simulink model "suspmod"  (Simulink 8.9)
settings: Solver=FixedStepAuto  StartTime=0.0  StopTime=50  FixedStep=0.01  RelTol=1e-3  AbsTol=1e-6
values from neighbouring files (symbols this model uses):
  m1 = 1    [fcn1.m]
  m2 = 1    [fcn1.m]
undefined symbols (not defined in the file or in its folder): b1, b2, k1, k2
settings Model: SuppressorTable=22 serialization::archive 11 0 6 0 0 0 11 0  Creator=Rick  LastModifiedBy=nikhil
settings DataIOCC: LimitDataPoints=off  SignalLoggingSaveFormat=Dataset
settings OptimizationCC: BlockReduction=off  BooleanDataType=off  ExpressionDepthLimit=2147483647
settings DebuggingCC: SaveWithParameterizedLinksMsg=none  SignalResolutionControl=TryResolveAllWithWarning  InheritedTsInSrcMsg=none  MultiTaskDSMMsg=warning  MultiTaskCondExecSysMsg=none  UnknownTsInhSupMsg=none
settings HardwareCC: TargetUnknown=on
settings GRTTargetCC: CombineOutputUpdateFcns=on  GRTInterface=off

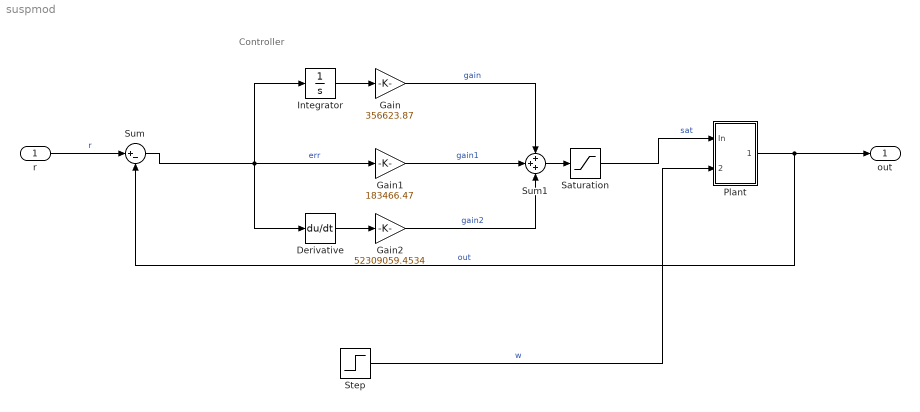
== system suspmod ==
  note: Controller
  r : Inport
  Derivative : Derivative
  Gain : Gain  Gain=356623.87
  Gain1 : Gain  Gain=183466.47
  Gain2 : Gain  Gain=52309059.4534
  Integrator : Integrator
  Plant : Subsystem
  Saturation : Saturate  UpperLimit=15  LowerLimit=-15
  Step : Step  Time=0  After=-.1  SampleTime=0
  Sum : Sum  Inputs=|+-
  Sum1 : Sum  Inputs=+++
  out : Outport
  wires:
  r/1 -> Sum/1  "r"
  Plant/1(Out) -> out/1, Sum/2  "out"
  Step/1 -> Plant/2(In1)  "w"
  Integrator/1 -> Gain/1
  Sum1/1 -> Saturation/1
  Sum/1 -> Derivative/1, Gain1/1, Integrator/1  "err"
  Gain1/1 -> Sum1/2  "gain1"
  Gain2/1 -> Sum1/3  "gain2"
  Saturation/1 -> Plant/1(In)  "sat"
  Derivative/1 -> Gain2/1
  Gain/1 -> Sum1/1  "gain"

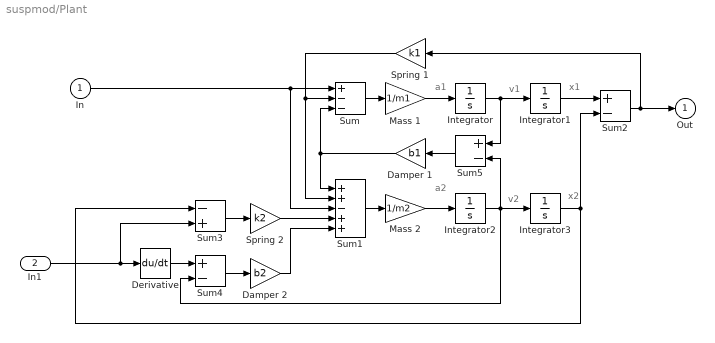
== system suspmod/Plant ==
  note: a1
  note: v1
  note: x1
  note: a2
  note: v2
  note: x2
  In : Inport
  In1 : Inport  Port=2
  Damper 1 : Gain  Gain=b1  SaturateOnIntegerOverflow=on  OutDataTypeStr=Inherit: Same as input  ParamDataTypeStr=Inherit: Same as input
  Damper 2 : Gain  Gain=b2  SaturateOnIntegerOverflow=on  OutDataTypeStr=Inherit: Same as input  ParamDataTypeStr=Inherit: Same as input
  Derivative : Derivative
  Integrator{,1..3} (4 alike) : Integrator
  Mass 1 : Gain  Gain=1/m1  SaturateOnIntegerOverflow=on  OutDataTypeStr=Inherit: Same as input  ParamDataTypeStr=Inherit: Same as input
  Mass 2 : Gain  Gain=1/m2  SaturateOnIntegerOverflow=on  OutDataTypeStr=Inherit: Same as input  ParamDataTypeStr=Inherit: Same as input
  Spring 1 : Gain  Gain=k1  SaturateOnIntegerOverflow=on  OutDataTypeStr=Inherit: Same as input  ParamDataTypeStr=Inherit: Same as input
  Spring 2 : Gain  Gain=k2  SaturateOnIntegerOverflow=on  OutDataTypeStr=Inherit: Same as input  ParamDataTypeStr=Inherit: Same as input
  Sum : Sum  Inputs=+--  SaturateOnIntegerOverflow=on  InputSameDT=on  OutDataTypeStr=Inherit: Same as first input
  Sum1 : Sum  Inputs=++-++  SaturateOnIntegerOverflow=on  InputSameDT=on  OutDataTypeStr=Inherit: Same as first input
  Sum2 : Sum  Inputs=+-  SaturateOnIntegerOverflow=on  InputSameDT=on  OutDataTypeStr=Inherit: Same as first input
  Sum3 : Sum  Inputs=-+  SaturateOnIntegerOverflow=on  InputSameDT=on  OutDataTypeStr=Inherit: Same as first input
  Sum4 : Sum  Inputs=+-  SaturateOnIntegerOverflow=on  InputSameDT=on  OutDataTypeStr=Inherit: Same as first input
  Sum5 : Sum  Inputs=+-  SaturateOnIntegerOverflow=on  InputSameDT=on  OutDataTypeStr=Inherit: Same as first input
  Out : Outport  InitialOutput=0
  wires:
  Sum5/1 -> Damper 1/1
  Derivative/1 -> Sum4/1
  Spring 1/1 -> Sum/2, Sum1/2
  Integrator3/1 -> Sum2/2, Sum3/1
  Sum3/1 -> Spring 2/1
  Integrator1/1 -> Sum2/1
  Damper 2/1 -> Sum1/5
  In/1 -> Sum/1, Sum1/3
  Mass 1/1 -> Integrator/1
  Sum1/1 -> Mass 2/1
  Integrator/1 -> Integrator1/1, Sum5/1
  In1/1 -> Sum3/2, Derivative/1
  Integrator2/1 -> Integrator3/1, Sum4/2, Sum5/2
  Spring 2/1 -> Sum1/4
  Mass 2/1 -> Integrator2/1
  Sum4/1 -> Damper 2/1
  Sum/1 -> Mass 1/1
  Damper 1/1 -> Sum1/1, Sum/3
  Sum2/1 -> Out/1, Spring 1/1
